simulink model "wlanhdlTimeAndFrequencySynchronization"  (R2025a)
settings: Solver=FixedStepDiscrete  StartTime=0.0  StopTime=stopTime  RelTol=1e-3
InitFcn:
  | wlanFrontEndInit;
values from neighbouring files (symbols this model uses):
  filterLatency = (wlanConfig.corrLen/filterUpsampleFactor)+filterUpsampleFactor+9    [wlanFrontEndInit.m]
  filterUpsampleFactor = 160e6/wlanConfig.Fs    [wlanFrontEndInit.m]
  Hd = dfilt.dffir(b)    [wlanFrontEndInit.m]
undefined symbols (not defined in the file or in its folder): Add, Shift, wlanConfig
libraries: simulink x14, hdlsllib x9, dspsrcs4 x3, dspsigops x3, dsphdlsigops2 x2, dsphdlmathfun2 x2, dsphdlfiltering2 x2
(part 2 of 2)

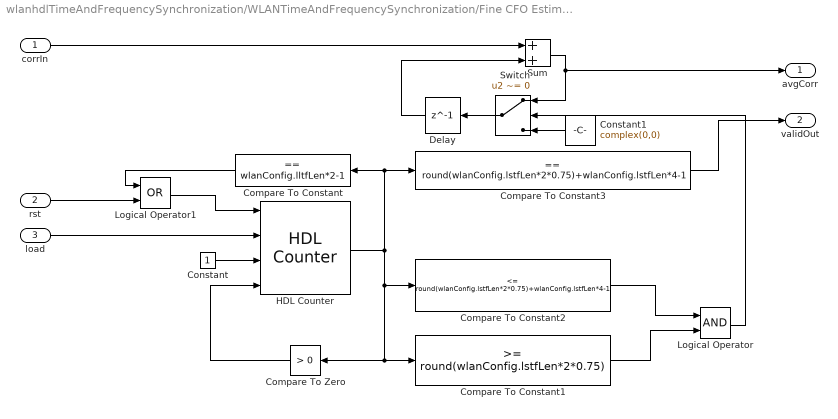
== system wlanhdlTimeAndFrequencySynchronization/WLANTimeAndFrequencySynchronization/Fine CFO Estimation and Correction/Fine CFO Estimation/Averager ==
  corrIn : Inport
  rst : Inport  Port=2
  load : Inport  Port=3
  Compare To Constant : simulink/Logic and Bit Operations/Compare To Constant  relop===  const=wlanConfig.lltfLen*2-1  OutDataTypeStr=boolean
      link override Compare: Operator===  OutDataTypeStr=boolean
  Compare To Constant1 : simulink/Logic and Bit Operations/Compare To Constant  relop=>=  const=round(wlanConfig.lstfLen*2*0.75)  OutDataTypeStr=boolean
      link override Compare: Operator=>=  OutDataTypeStr=boolean
  Compare To Constant2 : simulink/Logic and Bit Operations/Compare To Constant  relop=<=  const=round(wlanConfig.lstfLen*2*0.75)+wlanConfig.lstfLen*4-1  OutDataTypeStr=boolean
      link override Compare: Operator=<=  OutDataTypeStr=boolean
  Compare To Constant3 : simulink/Logic and Bit Operations/Compare To Constant  relop===  const=round(wlanConfig.lstfLen*2*0.75)+wlanConfig.lstfLen*4-1  OutDataTypeStr=boolean
      link override Compare: Operator===  OutDataTypeStr=boolean
  Compare To Zero : simulink/Logic and Bit Operations/Compare To Zero  relop=>  OutDataTypeStr=boolean
      link override Compare: Operator=>  OutDataTypeStr=boolean
  Constant : Constant  OutDataTypeStr=uint16  SampleTime=-1
  Constant1 : Constant  Value=complex(0,0)  OutDataTypeStr=Inherit: Inherit via back propagation  SampleTime=-1
  Delay : Delay  DelayLength=1
  HDL Counter : hdlsllib/Sources/HDL Counter  CountType=Count limited  CountInit=0  CountStep=1  CountMax=2*wlanConfig.lltfLen-1  CountFromType=Initial value  CountFrom=0  CountResetPort=on  CountLoadPort=on  CountEnbPort=on  CountDirPort=off  CountHitOutputPort=off  CountDataType=Unsigned  CountWordLen=16  CountFracLen=0  CountSampTime=1
      link override Add_wrap/Compare To Constant/Compare: Operator=>  OutDataTypeStr=boolean
      link override Sub_wrap/Compare To Constant/Compare: Operator=<  OutDataTypeStr=boolean
  Logical Operator : Logic  AllPortsSameDT=off  OutDataTypeStr=boolean
  Logical Operator1 : Logic  Operator=OR  AllPortsSameDT=off  OutDataTypeStr=boolean
  Sum : Sum  OutDataTypeStr=Inherit: Same as first input
  Switch : Switch  Criteria=u2 ~= 0  Threshold=1  SaturateOnIntegerOverflow=off  InputSameDT=off
  avgCorr : Outport
  validOut : Outport  Port=2
  wires:
  Constant/1 -> HDL Counter/3
  HDL Counter/1 -> Compare To Constant1/1, Compare To Zero/1, Compare To Constant2/1, Compare To Constant/1, Compare To Constant3/1
  Sum/1 -> avgCorr/1, Switch/1
  Compare To Zero/1 -> HDL Counter/4
  Compare To Constant1/1 -> Logical Operator/2
  rst/1 -> Logical Operator1/2
  Compare To Constant2/1 -> Logical Operator/1
  Constant1/1 -> Switch/3
  Logical Operator/1 -> Switch/2
  corrIn/1 -> Sum/1
  Switch/1 -> Delay/1
  Delay/1 -> Sum/2
  Compare To Constant/1 -> Logical Operator1/1
  Logical Operator1/1 -> HDL Counter/1
  load/1 -> HDL Counter/2
  Compare To Constant3/1 -> validOut/1

== system wlanhdlTimeAndFrequencySynchronization/WLANTimeAndFrequencySynchronization/Fine CFO Estimation and Correction/Fine CFO Estimation/Correlator ==
  dataIn : Inport
  Data Type Conversion : DataTypeConversion  OutDataTypeStr=fixdt(1,31,19)  SaturateOnIntegerOverflow=off  RndMeth=Floor
  Data Type Conversion1 : DataTypeConversion  OutDataTypeStr=fixdt(1,16,12)  SaturateOnIntegerOverflow=off  RndMeth=Floor
  Delay1 : Delay  InitialCondition=0  UseCircularBuffer=on
  Delay2 : Delay  DelayLength=wlanConfig.lstfLen*4  InitialCondition=0
  Delay3 : Delay  InitialCondition=0  UseCircularBuffer=on
  Delay32 : Delay  DelayLength=1
  Product : Product  RndMeth=Round
  complexConj : Math  Operator=conj  SignedPower=on  SaturateOnIntegerOverflow=off
  corrOut : Outport
  wires:
  Data Type Conversion/1 -> corrOut/1
  Delay1/1 -> Product/1
  Delay2/1 -> complexConj/1
  complexConj/1 -> Delay3/1
  Delay32/1 -> Data Type Conversion/1
  Data Type Conversion1/1 -> Delay1/1, Delay2/1
  Delay3/1 -> Product/2
  Product/1 -> Delay32/1
  dataIn/1 -> Data Type Conversion1/1

== system wlanhdlTimeAndFrequencySynchronization/WLANTimeAndFrequencySynchronization/Fine Time Sync/Correlator/MagnitudeSquared ==
  dataIn : Inport
  validIn : Inport  Port=2
  Add : Sum  OutDataTypeStr=Inherit: Same as accumulator
  Complex to Real-Imag : ComplexToRealImag
  Data Type Conversion : DataTypeConversion  OutDataTypeStr=fixdt(1,16,8)  SaturateOnIntegerOverflow=off  RndMeth=Floor
  Data Type Conversion1 : DataTypeConversion  OutDataTypeStr=fixdt(1,32,15)  SaturateOnIntegerOverflow=off  RndMeth=Floor
  Delay{,1..3} (4 alike) : Delay
  Delay4 : Delay  DelayLength=1
  Delay5 : Delay  DelayLength=1
  Delay6 : Delay  DelayLength=3
  Product1 : Product
  Product4 : Product
  dataOut : Outport  VectorParamsAs1DForOutWhenUnconnected=off
  validOut : Outport  Port=2  VectorParamsAs1DForOutWhenUnconnected=off
  wires:
  Complex to Real-Imag/2 -> Delay3/1, Delay2/1
  validIn/1 -> Delay6/1
  Complex to Real-Imag/1 -> Delay1/1, Delay/1
  Product4/1 -> Delay4/1
  Product1/1 -> Delay5/1
  Delay4/1 -> Add/1
  Delay5/1 -> Add/2
  Delay6/1 -> validOut/1
  dataIn/1 -> Data Type Conversion/1
  Delay1/1 -> Product4/2
  Delay2/1 -> Product1/1
  Delay3/1 -> Product1/2
  Delay/1 -> Product4/1
  Data Type Conversion/1 -> Complex to Real-Imag/1
  Data Type Conversion1/1 -> dataOut/1
  Add/1 -> Data Type Conversion1/1

== system wlanhdlTimeAndFrequencySynchronization/WLANTimeAndFrequencySynchronization/Fine Time Sync/Correlator/corrFilter ==
  note: delayLen=filterUpsampleFactor-1
  note: Latency = (coeffLen/filterUpsampleFactor)+filterUpsampleFactor+9
  dataIn : Inport
  validIn : Inport  Port=2
  rst : Inport  Port=3
  C1 : dsphdlfiltering2/Discrete FIR Filter  NumeratorSource=Property  Numerator=conj(flipud(wlanConfig.lltf(1:wlanConfig.corrLen))).'  NumeratorPrototype=[ 0.5, 0.5 ]  FilterStructure=Partly serial systolic  SerializationOption=Minimum number of cycles between valid input samples  NumCycles=filterUpsampleFactor  NumberOfMultipliers=2  SimulateUsing=Code generation  roundingMode=Floor  overflowMode=off  CoefficientsDataTypeStr=fixdt(1,16,14)  ResetInputPort=on  HDLGlobalReset=off  CoeffMultiplier=Multiplier  UseMultForPow2Coeff=on  FrameInputSymmOptim=off
  Delay : Delay  DelayLength=filterUpsampleFactor-1
  Delay1 : Delay  DelayLength=filterUpsampleFactor-1
  Delay2 : Delay  DelayLength=filterUpsampleFactor-1
  Downsample : DownSample  N=filterUpsampleFactor  RateOptions=Allow multirate processing
  Downsample1 : DownSample  N=filterUpsampleFactor  RateOptions=Allow multirate processing
  Terminator : Terminator
  Upsample : dspsigops/Upsample  FactorSource=Dialog parameter  N=filterUpsampleFactor  Nmax=16  phase=0  RateOptions=Allow multirate processing  ic=0  mode=Unused parameter value
  Upsample1 : dspsigops/Upsample  FactorSource=Dialog parameter  N=filterUpsampleFactor  Nmax=16  phase=0  RateOptions=Allow multirate processing  ic=0  mode=Unused parameter value
  Upsample2 : dspsigops/Upsample  FactorSource=Dialog parameter  N=filterUpsampleFactor  Nmax=16  phase=0  RateOptions=Allow multirate processing  ic=0  mode=Unused parameter value
  dataOut : Outport
  validOut : Outport  Port=2
  wires:
  dataIn/1 -> Upsample/1
  validIn/1 -> Upsample1/1
  Upsample1/1 -> C1/2
  C1/2 -> Delay1/1
  C1/3 -> Delay2/1
  Delay/1 -> Downsample/1
  Delay1/1 -> Downsample1/1
  Delay2/1 -> Terminator/1
  Downsample/1 -> dataOut/1
  Downsample1/1 -> validOut/1
  Upsample/1 -> C1/1
  C1/1 -> Delay/1
  rst/1 -> Upsample2/1
  Upsample2/1 -> C1/3

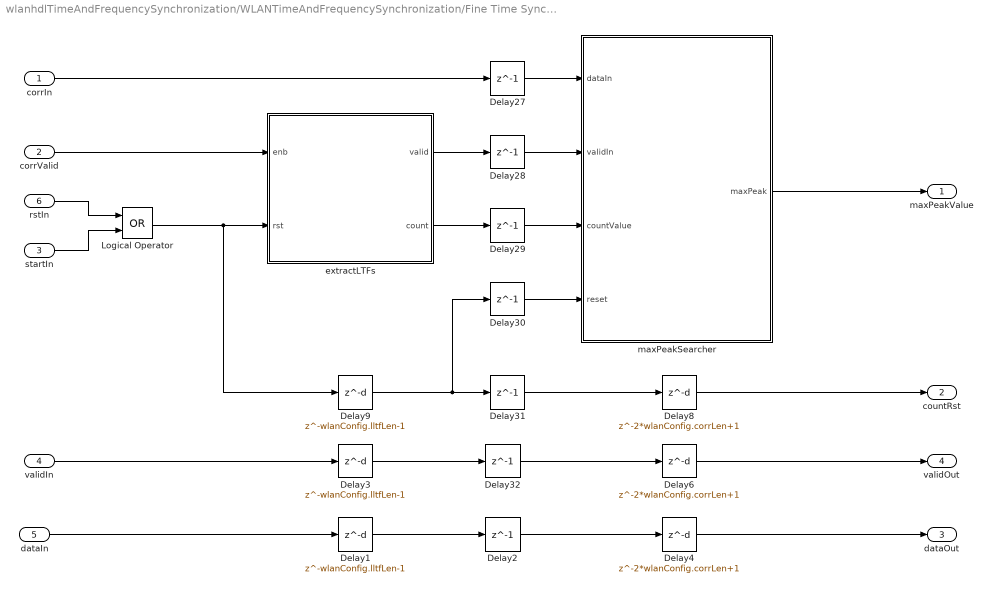
== system wlanhdlTimeAndFrequencySynchronization/WLANTimeAndFrequencySynchronization/Fine Time Sync/Peak Searcher/maxPeakSearcher ==
  corrIn : Inport
  corrValid : Inport  Port=2
  startIn : Inport  Port=3
  validIn : Inport  Port=4
  dataIn : Inport  Port=5
  rstIn : Inport  Port=6
  Delay1 : Delay  DelayLength=wlanConfig.lltfLen-1
  Delay{2,27..32} (7 alike) : Delay  DelayLength=1
  Delay3 : Delay  DelayLength=wlanConfig.lltfLen-1
  Delay4 : Delay  DelayLength=2*wlanConfig.corrLen+1
  Delay6 : Delay  DelayLength=2*wlanConfig.corrLen+1
  Delay8 : Delay  DelayLength=2*wlanConfig.corrLen+1
  Delay9 : Delay  DelayLength=wlanConfig.lltfLen-1
  Logical Operator : Logic  Operator=OR  AllPortsSameDT=off  OutDataTypeStr=boolean
  extractLTFs : Subsystem
  maxPeakSearcher : MATLAB Function  TreatAsAtomicUnit=on
  maxPeakValue : Outport
  countRst : Outport  Port=2
  dataOut : Outport  Port=3
  validOut : Outport  Port=4
  wires:
  Delay9/1 -> Delay31/1, Delay30/1
  Logical Operator/1 -> Delay9/1, extractLTFs/2(rst)
  extractLTFs/1(valid) -> Delay28/1
  Delay27/1 -> maxPeakSearcher/1(dataIn)
  Delay31/1 -> Delay8/1
  Delay30/1 -> maxPeakSearcher/4(reset)
  Delay29/1 -> maxPeakSearcher/3(countValue)
  extractLTFs/2(count) -> Delay29/1
  Delay28/1 -> maxPeakSearcher/2(validIn)
  maxPeakSearcher/1(maxPeak) -> maxPeakValue/1
  corrValid/1 -> extractLTFs/1(enb)
  corrIn/1 -> Delay27/1
  Delay32/1 -> Delay6/1
  Delay3/1 -> Delay32/1
  validIn/1 -> Delay3/1
  Delay6/1 -> validOut/1
  Delay2/1 -> Delay4/1
  Delay1/1 -> Delay2/1
  dataIn/1 -> Delay1/1
  Delay4/1 -> dataOut/1
  Delay8/1 -> countRst/1
  rstIn/1 -> Logical Operator/1
  startIn/1 -> Logical Operator/2

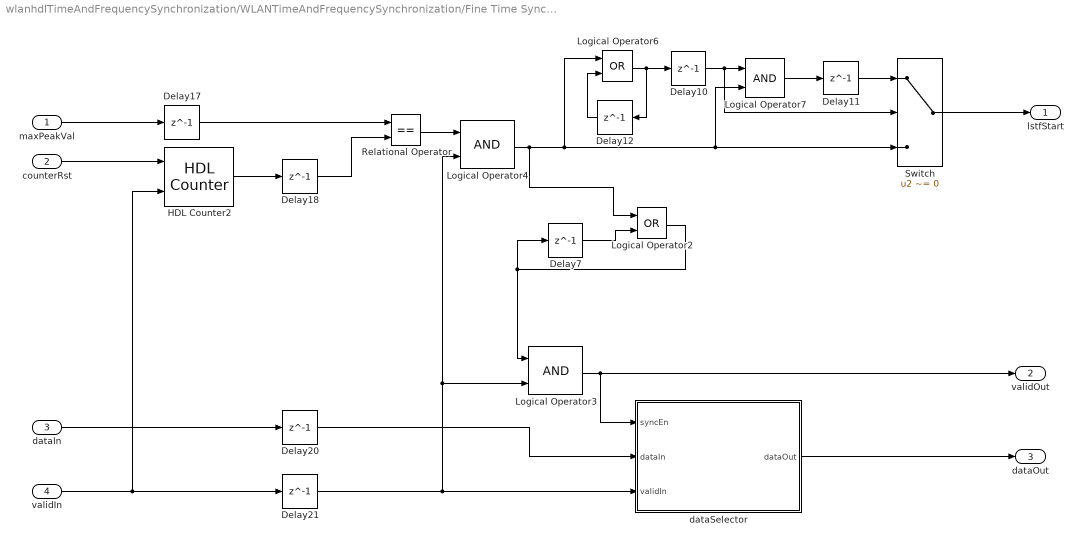
== system wlanhdlTimeAndFrequencySynchronization/WLANTimeAndFrequencySynchronization/Fine Time Sync/Peak Searcher/peakDetector ==
  maxPeakVal : Inport
  counterRst : Inport  Port=2
  dataIn : Inport  Port=3
  validIn : Inport  Port=4
  Delay{7,10..12,17..18,20..21} (8 alike) : Delay  DelayLength=1
  HDL Counter2 : hdlsllib/Sources/HDL Counter  CountType=Count limited  CountInit=0  CountStep=1  CountMax=2^16-1  CountFromType=Initial value  CountFrom=0  CountResetPort=on  CountLoadPort=off  CountEnbPort=on  CountDirPort=off  CountHitOutputPort=off  CountDataType=Unsigned  CountWordLen=16  CountFracLen=0  CountSampTime=1
      link override Add_wrap/Compare To Constant/Compare: Operator=>  OutDataTypeStr=boolean
      link override Sub_wrap/Compare To Constant/Compare: Operator=<  OutDataTypeStr=boolean
      link override const_load_val: OutDataTypeStr=fixdt(issigned,CountWordLen,CountFracLen,'DataTypeOverride','Off')
  Logical Operator2 : Logic  Operator=OR  AllPortsSameDT=off  OutDataTypeStr=boolean
  Logical Operator3 : Logic  AllPortsSameDT=off  OutDataTypeStr=boolean
  Logical Operator4 : Logic  AllPortsSameDT=off  OutDataTypeStr=boolean
  Logical Operator6 : Logic  Operator=OR  AllPortsSameDT=off  OutDataTypeStr=boolean
  Logical Operator7 : Logic  AllPortsSameDT=off  OutDataTypeStr=boolean
  Relational Operator : RelationalOperator  Operator===  OutDataTypeStr=boolean  RndMeth=Simplest  InputSameDT=off
  Switch : Switch  Criteria=u2 ~= 0  SaturateOnIntegerOverflow=off  InputSameDT=off
  "dataSelector " : MATLAB Function  TreatAsAtomicUnit=on
  lstfStart : Outport
  validOut : Outport  Port=2
  dataOut : Outport  Port=3
  wires:
  Relational Operator/1 -> Logical Operator4/1
  Logical Operator3/1 -> validOut/1, "dataSelector "/1(syncEn)
  Logical Operator6/1 -> Delay12/1, Delay10/1
  Logical Operator2/1 -> Delay7/1, Logical Operator3/1
  Delay21/1 -> "dataSelector "/3(validIn), Logical Operator3/2, Logical Operator4/2
  Delay10/1 -> Switch/2, Logical Operator7/1
  Delay7/1 -> Logical Operator2/2
  Delay17/1 -> Relational Operator/1
  Logical Operator4/1 -> Logical Operator2/1, Switch/3, Logical Operator7/2, Logical Operator6/1
  Delay11/1 -> Switch/1
  Delay20/1 -> "dataSelector "/2(dataIn)
  Delay12/1 -> Logical Operator6/2
  dataIn/1 -> Delay20/1
  "dataSelector "/1(dataOut) -> dataOut/1
  Logical Operator7/1 -> Delay11/1
  Delay18/1 -> Relational Operator/2
  HDL Counter2/1 -> Delay18/1
  maxPeakVal/1 -> Delay17/1
  Switch/1 -> lstfStart/1
  counterRst/1 -> HDL Counter2/1
  validIn/1 -> HDL Counter2/2, Delay21/1

== system wlanhdlTimeAndFrequencySynchronization/WLANTimeAndFrequencySynchronization/Coarse Time Sync/Correlator/MovingSum/Synchronous Enabled 128 Sample Delay  ==
  dataIn : Inport
  en : Inport  Port=2
  reset : Inport  Port=3
  Delay1 : Delay  DelayLength=wlanConfig.lstfLen  InitialCondition=0  ExternalReset=Level hold  ShowEnablePort=on
      settings: InputPortMap=u0,e6,r5
  State Control : StateControl  StateControl=Synchronous
  dataOut : Outport  VectorParamsAs1DForOutWhenUnconnected=off
  wires:
  en/1 -> Delay1/2
  dataIn/1 -> Delay1/1
  Delay1/1 -> dataOut/1
  reset/1 -> Delay1/3

== system wlanhdlTimeAndFrequencySynchronization/WLANTimeAndFrequencySynchronization/Coarse Time Sync/Energy Calculator/magnitudeSquared/MagnitudeSquared ==
  dataIn : Inport
  validIn : Inport  Port=2
  Add : Sum  OutDataTypeStr=Inherit: Same as accumulator
  Complex to Real-Imag : ComplexToRealImag
  DTadjust : MATLAB Function  TreatAsAtomicUnit=on
  Delay{,1..3} (4 alike) : Delay
  Delay4 : Delay  DelayLength=1
  Delay5 : Delay  DelayLength=1
  Delay6 : Delay  DelayLength=3
  Product1 : Product
  Product4 : Product
  dataOut : Outport  VectorParamsAs1DForOutWhenUnconnected=off
  validOut : Outport  Port=2  VectorParamsAs1DForOutWhenUnconnected=off
  wires:
  Complex to Real-Imag/2 -> Delay3/1, Delay2/1
  dataIn/1 -> Complex to Real-Imag/1
  validIn/1 -> Delay6/1
  Complex to Real-Imag/1 -> Delay1/1, Delay/1
  Product4/1 -> Delay4/1
  Product1/1 -> Delay5/1
  Delay/1 -> Product4/2
  Delay1/1 -> Product4/1
  Delay2/1 -> Product1/1
  Delay3/1 -> Product1/2
  Delay4/1 -> Add/1
  Delay5/1 -> Add/2
  Delay6/1 -> validOut/1
  Add/1 -> DTadjust/1(in)
  DTadjust/1(out) -> dataOut/1

== system wlanhdlTimeAndFrequencySynchronization/WLANTimeAndFrequencySynchronization/Coarse Time Sync/Energy Calculator/magnitudeSquared/MagnitudeSquared1 ==
  dataIn : Inport
  validIn : Inport  Port=2
  Add : Sum  OutDataTypeStr=Inherit: Same as accumulator
  Complex to Real-Imag : ComplexToRealImag
  Delay{,1..3} (4 alike) : Delay
  Delay4 : Delay  DelayLength=1
  Delay5 : Delay  DelayLength=1
  Delay6 : Delay  DelayLength=3
  Product1 : Product
  Product4 : Product
  dataOut : Outport  VectorParamsAs1DForOutWhenUnconnected=off
  validOut : Outport  Port=2  VectorParamsAs1DForOutWhenUnconnected=off
  wires:
  Complex to Real-Imag/2 -> Delay3/1, Delay2/1
  dataIn/1 -> Complex to Real-Imag/1
  validIn/1 -> Delay6/1
  Complex to Real-Imag/1 -> Delay1/1, Delay/1
  Product4/1 -> Delay4/1
  Product1/1 -> Delay5/1
  Add/1 -> dataOut/1
  Delay/1 -> Product4/2
  Delay1/1 -> Product4/1
  Delay2/1 -> Product1/1
  Delay3/1 -> Product1/2
  Delay4/1 -> Add/1
  Delay5/1 -> Add/2
  Delay6/1 -> validOut/1

== system wlanhdlTimeAndFrequencySynchronization/WLANTimeAndFrequencySynchronization/Coarse Time Sync/Energy Calculator/magnitudeSquared/MovingSum ==
  dataIn : Inport
  validIn : Inport  Port=2
  Add : Sum  Inputs=|+-  OutDataTypeStr=Inherit: Same as accumulator
  Add1 : Sum  Inputs=|++  OutDataTypeStr=Inherit: Same as accumulator
  Delay{3..6,12} (5 alike) : Delay  DelayLength=1  InitialCondition=0
  Shift Arithmetic : ArithShift  BitShiftNumber=1  BitShiftDirection=Right
  "Synchronous Enabled 16 Sample Delay " : Subsystem
  Synchronous Enabled Unit Delay : hdlsllib/Discrete/Unit Delay Enabled Synchronous  InitialCondition=0.0  SampleTime=-1
  dataOut : Outport  VectorParamsAs1DForOutWhenUnconnected=off
  validOut : Outport  Port=2  VectorParamsAs1DForOutWhenUnconnected=off
  wires:
  "Synchronous Enabled 16 Sample Delay "/1(dataOut) -> Add/2
  Synchronous Enabled Unit Delay/1 -> Delay5/1, Add1/2
  dataIn/1 -> Add/1, "Synchronous Enabled 16 Sample Delay "/1(dataIn)
  Delay6/1 -> validOut/1
  Delay5/1 -> dataOut/1
  Delay4/1 -> Delay6/1
  Delay3/1 -> Delay4/1, Synchronous Enabled Unit Delay/2
  Delay12/1 -> Add1/1
  validIn/1 -> Delay3/1, "Synchronous Enabled 16 Sample Delay "/2(en)
  Add/1 -> Shift Arithmetic/1
  Add1/1 -> Synchronous Enabled Unit Delay/1
  Shift Arithmetic/1 -> Delay12/1

== system wlanhdlTimeAndFrequencySynchronization/WLANTimeAndFrequencySynchronization/Fine Time Sync/Peak Searcher/maxPeakSearcher/extractLTFs ==
  enb : Inport
  rst : Inport  Port=2
  Compare To Constant : simulink/Logic and Bit Operations/Compare To Constant  relop=>=  const=length(wlanConfig.lltf)-1  OutDataTypeStr=boolean
      link override Compare: Operator=>=  OutDataTypeStr=boolean
  Compare To Constant1 : simulink/Logic and Bit Operations/Compare To Constant  relop=<  const=wlanConfig.corrLen*2+1  OutDataTypeStr=boolean
      link override Compare: Operator=<  OutDataTypeStr=boolean
  HDL Counter : hdlsllib/Sources/HDL Counter  CountType=Count limited  CountInit=0  CountStep=1  CountMax=2^16-1  CountFromType=Initial value  CountFrom=0  CountResetPort=on  CountLoadPort=off  CountEnbPort=on  CountDirPort=off  CountHitOutputPort=off  CountDataType=Unsigned  CountWordLen=16  CountFracLen=0  CountSampTime=1
      link override Add_wrap/Compare To Constant/Compare: Operator=>  OutDataTypeStr=boolean
      link override Sub_wrap/Compare To Constant/Compare: Operator=<  OutDataTypeStr=boolean
      link override const_load_val: OutDataTypeStr=fixdt(issigned,CountWordLen,CountFracLen,'DataTypeOverride','Off')
  HDL Counter1 : hdlsllib/Sources/HDL Counter  CountType=Count limited  CountInit=0  CountStep=1  CountMax=2^16-1  CountFromType=Initial value  CountFrom=0  CountResetPort=on  CountLoadPort=off  CountEnbPort=on  CountDirPort=off  CountHitOutputPort=off  CountDataType=Unsigned  CountWordLen=16  CountFracLen=0  CountSampTime=1
      link override Add_wrap/Compare To Constant/Compare: Operator=>  OutDataTypeStr=boolean
      link override Sub_wrap/Compare To Constant/Compare: Operator=<  OutDataTypeStr=boolean
      link override const_load_val: OutDataTypeStr=fixdt(issigned,CountWordLen,CountFracLen,'DataTypeOverride','Off')
  Logical Operator : Logic  AllPortsSameDT=off  OutDataTypeStr=boolean
  Logical Operator1 : Logic  AllPortsSameDT=off  OutDataTypeStr=boolean
  valid : Outport
  count : Outport  Port=2
  wires:
  Compare To Constant1/1 -> Logical Operator1/1
  Logical Operator/1 -> Logical Operator1/2, HDL Counter1/2
  enb/1 -> Logical Operator/2, HDL Counter/2
  Logical Operator1/1 -> valid/1
  HDL Counter/1 -> Compare To Constant/1
  Compare To Constant/1 -> Logical Operator/1
  rst/1 -> HDL Counter1/1, HDL Counter/1
  HDL Counter1/1 -> count/1, Compare To Constant1/1

== system wlanhdlTimeAndFrequencySynchronization/WLANTimeAndFrequencySynchronization/Coarse Time Sync/Energy Calculator/magnitudeSquared/MovingSum/Synchronous Enabled 16 Sample Delay  ==
  dataIn : Inport
  en : Inport  Port=2
  Delay1 : Delay  DelayLength=wlanConfig.lstfLen  InitialCondition=0  ShowEnablePort=on
      settings: InputPortMap=u0,e6
  State Control : StateControl  StateControl=Synchronous
  dataOut : Outport  VectorParamsAs1DForOutWhenUnconnected=off
  wires:
  en/1 -> Delay1/2
  dataIn/1 -> Delay1/1
  Delay1/1 -> dataOut/1

== matlab function wlanhdlTimeAndFrequencySynchronization/WLANTimeAndFrequencySynchronization/Coarse Time Sync/Peak Detector/searchStartOfFrame ==
  data: thresholdValid input; valid input; syncOut output; wlanConfig parameter
function syncOut  = searchStartOfFrame(thresholdValid,valid,wlanConfig)
%#codegen
persistent countVal;
persistent countEnb;
persistent validCount;
persistent detectFlag;
persistent detectFlagCount;

WL = ceil(log2(wlanConfig.lstfLen*10));
if isempty(countVal)
    countVal = fi(0,0,WL,0);
    countEnb = false;
end
if isempty(detectFlag)
    detectFlag = false;
    detectFlagCount = fi(0,0,WL,0);
end
if isempty(validCount)
    validCount = fi(0,0,WL,0); % Considering max count of 10 for STFs
end
if valid && thresholdValid 
    validCount(:) = validCount + 1;
    countEnb = true;
end
if detectFlagCount > 0
    detectFlagCount(:) = detectFlagCount+1;
end
if countEnb
    countVal(:) = countVal + 1;
    if countVal == wlanConfig.lstfLen*10+1
        countVal(:) = 0;
        countEnb = false;
        if validCount > wlanConfig.lstfLen*5
            detectFlag = true;
            detectFlagCount(:) =1;
        else
            detectFlag = false;
        end
        validCount(:) = 0;
    end
end

if detectFlagCount > wlanConfig.lstfLen*10
    detectFlagCount(:)=0;
    detectFlag = false;
end
syncOut = detectFlag;

== matlab function wlanhdlTimeAndFrequencySynchronization/WLANTimeAndFrequencySynchronization/Coarse Time Sync/Stream Synchronizer/StreamSyncronizer ==
  data: pop input; dataIn input; dataOut output; push input; validOut output; depth parameter
function [dataOut, validOut] = SynchronousFIFO(pop,dataIn,push,depth)
    %#codegen
    
    coder.extrinsic('warning');
    coder.extrinsic('num2str');
    
    persistent wrAddr rdAddr dataOutReg validOutReg mem mem1 mem2 level;
    
    %------------------------------------------------------------------------
    % Constants
    %------------------------------------------------------------------------
    
    addrWL = nextpow2(depth);
    
    %------------------------------------------------------------------------
    % Persistent variable initialization
    %------------------------------------------------------------------------
    
    if isempty(mem)
        
        wrAddr      = fi(0,0,addrWL,0,hdlfimath);
        rdAddr      = fi(0,0,addrWL,0,hdlfimath);
        dataOutReg  = cast(0,'like',dataIn);
        validOutReg = false;
        mem         = zeros(depth,1,'like',dataIn);
        mem1         = zeros(depth,1,'like',dataIn);
        mem2         = zeros(depth,1,'like',dataIn);
        % For generating warnings only. Not for code gen.
        level       = int16(0);
                
    end
    
    %------------------------------------------------------------------------
    % Outputs
    %------------------------------------------------------------------------
    
    dataOut  = dataOutReg;
    validOut = validOutReg;
    
    %------------------------------------------------------------------------
    % Calculate next state values
    %------------------------------------------------------------------------
    
    if pop
        
        dataOutReg(:) = mem(rdAddr+1);
        rdAddr(:)     = rdAddr+1;
        level(:)      = level-1;
        
        if level < 0
            warning('Buffer underflow: attempt to pop data out of empty buffer.');
        end
        
    end
    
    if push
        
        mem(wrAddr+1) = dataIn;
        wrAddr(:)     = wrAddr+1;
        level(:)      = level+1;
        
        if level > depth            
            warning(['Buffer overflow: attempt to push data into full buffer. Level = ', num2str(level), '.']);
        end
        
    end
    
    validOutReg = pop;
    
end

== matlab function wlanhdlTimeAndFrequencySynchronization/WLANTimeAndFrequencySynchronization/Rx Filter/DTConverter ==
  data: dataIn1 input; dataOut output; dataIn2 input
function dataOut = DTConverter(dataIn1,dataIn2)
%#codegen
dataOut = cast(dataIn2,'like',dataIn1);
end

== matlab function wlanhdlTimeAndFrequencySynchronization/WLANTimeAndFrequencySynchronization/Coarse CFO Estimation and Correction/Coarse CFO Correction/DTConverter ==
  data: dataIn1 input; dataOut output; dataIn2 input
function dataOut = DTConverter(dataIn1,dataIn2)
%#codegen
dataOut = cast(dataIn2,'like',dataIn1);
end

== matlab function wlanhdlTimeAndFrequencySynchronization/WLANTimeAndFrequencySynchronization/Fine CFO Estimation and Correction/Fine CFO Correction/DTConverter ==
  data: dataIn1 input; dataOut output; dataIn2 input
function dataOut = DTConverter(dataIn1,dataIn2)
%#codegen
dataOut = cast(dataIn2,'like',dataIn1);
end

== matlab function wlanhdlTimeAndFrequencySynchronization/WLANTimeAndFrequencySynchronization/Coarse Time Sync/Correlator/delayedCorrelation/DTadjust ==
  data: in input; out output; wlanConfig parameter
function out = DTadjust(in,wlanConfig)
%#codegen
if isfloat(in)
    out = in;
else
    WL = in.WordLength;
    FL = WL - (log2(wlanConfig.lstfLen)+1)-1;
    out = fi(in,1,WL,FL);
end

== matlab function wlanhdlTimeAndFrequencySynchronization/WLANTimeAndFrequencySynchronization/Coarse Time Sync/Energy Calculator/magnitudeSquared/MagnitudeSquared/DTadjust ==
  data: in input; out output; wlanConfig parameter
function out = DTadjust(in,wlanConfig)
%#codegen
if isfloat(in)
    out = in;
else
    WL = in.WordLength;
    FL = WL - (log2(wlanConfig.lstfLen)+1)-1;
    out = fi(in,1,WL,FL);
end

== matlab function wlanhdlTimeAndFrequencySynchronization/WLANTimeAndFrequencySynchronization/Coarse CFO Estimation and Correction/Coarse CFO Estimation/Sample FreqOff ==
  data: freqOffIn input; freqOffOut output; enb input; rst input
function freqOffOut = sampleFreqOff(freqOffIn,enb,rst)
%#codegen

persistent freqReg;
persistent freqFlag;

if isempty(freqReg)||rst
    freqReg = cast(0,'like',freqOffIn);
    freqFlag = true;
end

if enb && freqFlag   
        freqReg = freqOffIn;
        freqFlag = false;      
end

freqOffOut = freqReg;

== matlab function wlanhdlTimeAndFrequencySynchronization/WLANTimeAndFrequencySynchronization/Fine CFO Estimation and Correction/Fine CFO Estimation/sample FreqOff ==
  data: freqOffIn input; freqOffOut output; enb input; rst input
function freqOffOut = sampleFreqOff(freqOffIn,enb,rst)
%#codegen

persistent freqReg;
persistent freqFlag;

if isempty(freqReg)||rst
    freqReg = cast(0,'like',freqOffIn);
    freqFlag = true;
end

if enb && freqFlag   
        freqReg = freqOffIn;
        freqFlag = false;      
end

freqOffOut = freqReg;

== matlab function wlanhdlTimeAndFrequencySynchronization/WLANTimeAndFrequencySynchronization/Fine Time Sync/Peak Searcher/maxPeakSearcher/maxPeakSearcher ==
  data: dataIn input; maxPeak output; validIn input; countValue input; reset input; wlanConfig parameter
function maxPeak  = maxPeakSearcher(dataIn,validIn,countValue,reset,wlanConfig)
%#codegen

persistent maxPeakReg;
persistent maxPeakPrev;
persistent maxValueReg;

if isempty(maxPeakReg) || reset
    maxValueReg = cast(0,'like',dataIn);
    maxPeakReg = cast(0,'like',countValue);
    maxPeakPrev = cast(0,'like',countValue);
end

if validIn
    if dataIn > maxValueReg        
       maxPeakReg = countValue;
       maxValueReg = dataIn;
    end
end

if countValue == 2*wlanConfig.corrLen-1
    maxPeak  = maxPeakReg-wlanConfig.corrLen;
    maxPeakPrev = maxPeak;
else
    maxPeak  = cast(maxPeakPrev,'like',countValue);
end

== matlab function wlanhdlTimeAndFrequencySynchronization/WLANTimeAndFrequencySynchronization/Fine Time Sync/Peak Searcher/peakDetector/dataSelector  ==
  data: syncEn input; dataIn input; dataOut output; validIn input
function dataOut = dataSelector(syncEn,dataIn,validIn)
%#codegen

if validIn && syncEn
    dataOut = dataIn;
else
    dataOut = cast(complex(0,0),'like',dataIn);
end

== matlab function wlanhdlTimeAndFrequencySynchronization/WLANTimeAndFrequencySynchronization/Coarse Time Sync/Energy Calculator/streamSynchronizer/StreamSyncronizer ==
  data: pop input; dataIn input; dataOut output; push input; validOut output; depth parameter
function [dataOut, validOut] = SynchronousFIFO(pop,dataIn,push,depth)
    %#codegen
    
    coder.extrinsic('warning');
    coder.extrinsic('num2str');
    
    persistent wrAddr rdAddr dataOutReg validOutReg mem level;
    
    %------------------------------------------------------------------------
    % Constants
    %------------------------------------------------------------------------
    
    addrWL = nextpow2(depth);
    
    %------------------------------------------------------------------------
    % Persistent variable initialization
    %------------------------------------------------------------------------
    
    if isempty(mem)
        
        wrAddr      = fi(0,0,addrWL,0,hdlfimath);
        rdAddr      = fi(0,0,addrWL,0,hdlfimath);
        dataOutReg  = cast(0,'like',dataIn);
        validOutReg = false;
        mem         = zeros(depth,1,'like',dataIn);
        % For generating warnings only. Not for code gen.
        level       = int16(0);
                
    end
    
    %------------------------------------------------------------------------
    % Outputs
    %------------------------------------------------------------------------
    
    dataOut  = dataOutReg;
    validOut = validOutReg;
    
    %------------------------------------------------------------------------
    % Calculate next state values
    %------------------------------------------------------------------------
    
    if pop
        
        dataOutReg(:) = mem(rdAddr+1);
        rdAddr(:)     = rdAddr+1;
        level(:)      = level-1;
        
        if level < 0
            warning('Buffer underflow: attempt to pop data out of empty buffer.');
        end
        
    end
    
    if push
        
        mem(wrAddr+1) = dataIn;
        wrAddr(:)     = wrAddr+1;
        level(:)      = level+1;
        
        if level > depth            
            warning(['Buffer overflow: attempt to push data into full buffer. Level = ', num2str(level), '.']);
        end
        
    end
    
    validOutReg = pop;
    
end

== matlab function wlanhdlTimeAndFrequencySynchronization/WLANTimeAndFrequencySynchronization/Coarse Time Sync/Peak Detector/MATLAB Function1 ==
  data: syncEn input; dataIn input; dataOut output; validIn input
function dataOut = dataSelector(syncEn,dataIn,validIn)
%#codegen

if validIn && syncEn
    dataOut = dataIn;
else
    dataOut = cast(complex(0,0),'like',dataIn);
end
